simulink library "lib_conversion"  (R2023a)
settings: Solver=VariableStepAuto  StartTime=0.0  StopTime=10.0  RelTol=1e-3
settings Model: Creator=cav2ofo  LastModifiedBy=lenovo
settings OptimizationCC: ReuseModelBlockBuffer=off

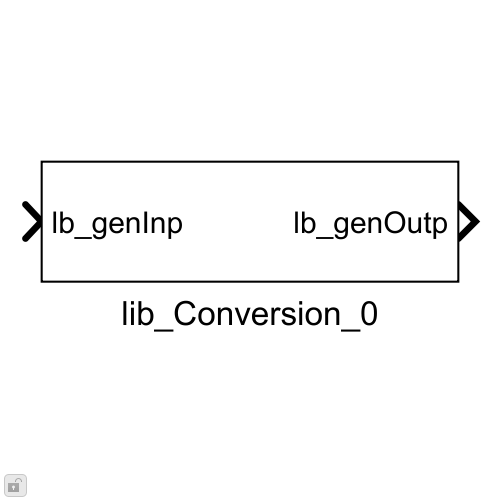
[thumbnail: Simulink's stored preview of the top-level diagram]
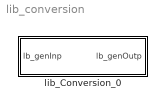
== system lib_conversion ==
  lib_Conversion_0 : Subsystem  mask{lb_parDataType=Inherit: Inherit via back propagation, lb_parOutpMaxVal=[], lb_parOutpMinVal=[], RndMeth=Floor, lb_parSatFlag=off}
      mask prompts: lb_parDataType "Data type:"; lb_parOutpMaxVal "Output maximum value:"; lb_parOutpMinVal "Output minimum value:"; RndMeth "Simulink:blkprm_prompts:SPP_RndMeth_ID"; lb_parSatFlag "Simulink:blkprm_prompts:AllBlksSaturate"
      mask init:
      | if not(isobject(lb_parDataType))
      |     lb_parIntDataType = lb_parDataType;
      | else
      |     if strcmp(lb_parDataType.DataTypeMode,'Fixed-point: unspecified scaling')
      |         if strcmp(lb_parDataType.Signedness,'Signed')
      |             temp.dataType = fi([lb_parOutpMinVal,lb_parOutpMaxVal],1,...
      |                 lb_parDataType.WordLength);
      |         else
      |             temp.dataType = fi([lb_parOutpMinVal,lb_parOutpMaxVal],0,...
      |             lb_parDataType.WordLength);
      |         end
      |         lb_parIntDataType = Simulink.NumericType;
      |         lb_parIntDataType.DataTypeMode = 'Fixed-point: slope and bias scaling';
      |         lb_parIntDataType.Signedness = temp.dataType.Signedness;
      |         lb_parIntDataType.WordLength = temp.dataType.WordLength;
      |         lb_parIntDataType.Slope = 2^-(temp.dataType.FractionLength);
      |     else
      |         lb_parIntDataType = lb_parDataType;
      |     end
      | end
      mask TypeOptions RndMeth: Data Type Conversion/RndMeth
      mask TypeOptions lb_parSatFlag: Data Type Conversion/SaturateOnIntegerOverflow
      mask DialogControl DescGroupVar Prompt: VHIT control library
      mask DialogControl DescTextVar Prompt: Data type conversion and duplicate
      mask DialogControl RndMeth Prompt: 整数舍入模式:
      mask DialogControl lb_parSatFlag Prompt: 对整数溢出进行饱和处理

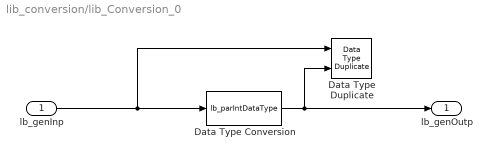
== system lib_conversion/lib_Conversion_0 ==
  lb_genInp : Inport
  Data Type Duplicate : DataTypeDuplicate
  Data Type Conversion : DataTypeConversion  OutDataTypeStr=lb_parIntDataType  SaturateOnIntegerOverflow=off  RndMeth=Floor
  lb_genOutp : Outport
  wires:
  Data Type Conversion/1 -> Data Type Duplicate/2, lb_genOutp/1
  lb_genInp/1 -> Data Type Duplicate/1, Data Type Conversion/1
